simulink model "F250Main"  (R2020b)
settings: Solver=ode8  StartTime=0.0  StopTime=10  FixedStep=0.001  RelTol=1e-3
model workspace: external: MATLAB File C:\Users\zxz\Desktop\matlab\m2020b\F250SimGithub\F250Main_DataFile.m (data not in the file)
values from neighbouring files (symbols this model uses):
  FData = [ 5.1001, ... (first row only)    [F250Main_DataFile.m]
  m = 1.13    [F250Main_DataFile.m]
  PWMData = 0.5:0.05:1    [F250Main_DataFile.m]
undefined symbols (not defined in the file or in its folder): smiData, X, Y, Z
libraries: sm_lib x125, nesl_utility x36, aerolibconvert2 x13, sharedtransform x1
(part 1 of 3)
settings Model: Creator=zxz  LastModifiedBy=zxz

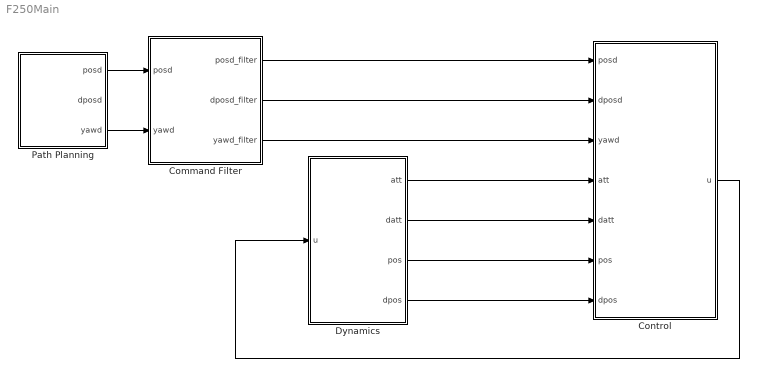
== system F250Main ==
  Command Filter : Subsystem
  Control : Subsystem
  Dynamics : Subsystem
  Path Planning : Subsystem
  wires:
  Path Planning/1(posd) -> Command Filter/1(posd)
  Path Planning/3(yawd) -> Command Filter/2(yawd)
  Control/1(u) -> Dynamics/1(u)
  Command Filter/1(posd_filter) -> Control/1(posd)
  Command Filter/2(dposd_filter) -> Control/2(dposd)
  Command Filter/3(yawd_filter) -> Control/3(yawd)
  Dynamics/1(att) -> Control/4(att)
  Dynamics/2(datt) -> Control/5(datt)
  Dynamics/3(pos) -> Control/6(pos)
  Dynamics/4(dpos) -> Control/7(dpos)

== system F250Main/Command Filter ==
  posd : Inport
  yawd : Inport  Port=2
  Demux11 : Demux  Outputs=3
  Mux1 : Mux  Inputs=3
  Mux8 : Mux  Inputs=3
  X Channel : Subsystem
  Y Channel : Subsystem
  Yaw Channel : Subsystem
  Z Channel : Subsystem
  posd_filter : Outport  VectorParamsAs1DForOutWhenUnconnected=off
  dposd_filter : Outport  Port=2  VectorParamsAs1DForOutWhenUnconnected=off
  yawd_filter : Outport  Port=3  VectorParamsAs1DForOutWhenUnconnected=off
  wires:
  yawd/1 -> Yaw Channel/1(yawd)
  posd/1 -> Demux11/1
  Demux11/1 -> X Channel/1(xd)
  Demux11/2 -> Y Channel/1(yd)
  Demux11/3 -> Z Channel/1(zd)
  Yaw Channel/1(zd_filter) -> yawd_filter/1
  Mux8/1 -> posd_filter/1
  X Channel/1(xd_filter) -> Mux8/1
  Y Channel/1(yd_filter) -> Mux8/2
  Z Channel/1(zd_filter) -> Mux8/3
  X Channel/2(dxd_filter) -> Mux1/1
  Y Channel/2(dyd_filter) -> Mux1/2
  Z Channel/2(dzd_filter) -> Mux1/3
  Mux1/1 -> dposd_filter/1

== system F250Main/Control ==
  posd : Inport
  dposd : Inport  Port=2
  yawd : Inport  Port=3
  att : Inport  Port=4
  datt : Inport  Port=5
  pos : Inport  Port=6
  dpos : Inport  Port=7
  Cascade Attitude Control : Subsystem
  Mux : Mux
  Mux1 : Mux  Inputs=3
  Position Control : Subsystem
  u : Outport  VectorParamsAs1DForOutWhenUnconnected=off
  wires:
  Mux/1 -> u/1
  att/1 -> Position Control/5(att), Cascade Attitude Control/2(att)
  datt/1 -> Cascade Attitude Control/3(datt)
  Mux1/1 -> Cascade Attitude Control/1(attd)
  yawd/1 -> Mux1/3
  Cascade Attitude Control/1(u2) -> Mux/2
  Cascade Attitude Control/2(u3) -> Mux/3
  Cascade Attitude Control/3(u4) -> Mux/4
  posd/1 -> Position Control/1(posd)
  dposd/1 -> Position Control/2(dposd)
  pos/1 -> Position Control/3(pos)
  dpos/1 -> Position Control/4(dpos)
  Position Control/1(u1) -> Mux/1
  Position Control/2(rolld) -> Mux1/1
  Position Control/3(pitchd) -> Mux1/2

== system F250Main/Dynamics ==
  u : Inport
  Infinite Plane : sm_lib/Curves and Surfaces/Infinite Plane  GraphicType=Rectangle  GraphicPlaneWidth=5  GraphicPlaneWidthUnits=m  GraphicPlaneHeight=5  GraphicPlaneHeightUnits=m  GraphicVisPropType=SimpleVisualProperties  GraphicDiffuseColor=[0.5 0.5 0.5]  GraphicOpacity=0.25  GraphicSpecularColor=[0.5 0.5 0.5 1.0]  GraphicAmbientColor=[0.15 0.15 0.15 1.0]  GraphicEmissiveColor=[0.0 0.0 0.0 1.0]  GraphicShininess=75
  MechanismConfiguration : sm_lib/Utilities/Mechanism Configuration  UniformGravity=Constant  GravityVector=[0 0 -9.81]  GravityVectorUnits=m/s^2  GravityUnits=m/s^2  LinearizationDelta=0.001  JointModeTransitionNonlinearIterations=2
  Rigid Transform : sm_lib/Frames and Transforms/Rigid Transform  TranslationMethod=Cartesian  TranslationStandardOffset=0  TranslationLengthUnit=m  TranslationStandardAxis=+Z  TranslationCartesianOffset=[0 0 -0.5]  TranslationROffset=0  TranslationROffsetUnits=m  TranslationZOffset=0  TranslationZOffsetUnits=m  TranslationThetaOffset=0  TranslationThetaOffsetUnits=deg  RotationMethod=None  RotationAngleUnits=deg  RotationStandardAxis=+Z  RotationAngle=0.0  RotationArbitraryAxis=[0 0 1]  FollAlignAxisA=+X  BaseAlignAxisA=+Y  FollAlignAxisB=+Y  BaseAlignAxisB=+Z  RotationSequenceAxes=FollowerAxes  RotationSequence=XYX  RotationSequenceAngles=[0 0 0]  RotationSequenceAnglesUnits=deg  RotationMatrix=[1 0 0; 0 1 0; 0 0 1]
  Solver Configuration : nesl_utility/Solver Configuration  PhysicalDomain=network_engine_domain  SubClassName=solver  LeftPortType=input  RightPortType=generic  Tones=[]  Harmonics=[]  SimulateNoise=off  Profile=off  UseLocalSampling=off  EnableSwitchedLinearOptims=on  FrequencyDomain=off  UseCCode=off  RelTol=0.001  AbsTol=1e-06  MinStep=1e-09  ToWorkspace=off  RevertToSquareIcSolve=off  NumHomotopyIterations=100  PhasorMode=off  PhasorModeNumHarmonics=1  DoDC=off  ResidualTolerance=1e-09  UseLocalSolver=off  LocalSolverChoice=NE_BACKWARD_EULER_ADVANCER  LocalSolverSampleTime=0.001  DoFixedCost=off  MaxNonlinIter=3  MaxModeIter=2  ComputeImpulses=off  ImpulseIterations=2  LinearAlgebra=auto  EquationFormulation=NE_TIME_EF  DelaysMemoryBudget=1024  AutomaticFiltering=on  FilteringTimeConstant=0.001  PartitionStorageMethod=AS_NEEDED  PartitionMemoryBudget=1024  PartitionMethod=ROBUST
  Subsystem : Subsystem
  Transform : sm_lib/Frames and Transforms/Rigid Transform  TranslationMethod=Cartesian  TranslationStandardOffset=0  TranslationLengthUnit=mm  TranslationStandardAxis=+Z  TranslationCartesianOffset=smiData.RigidTransform(4).translation  TranslationROffset=0  TranslationROffsetUnits=m  TranslationZOffset=0  TranslationZOffsetUnits=m  TranslationThetaOffset=0  TranslationThetaOffsetUnits=deg  RotationMethod=ArbitraryAxis  RotationAngleUnits=rad  RotationStandardAxis=+Z  RotationAngle=smiData.RigidTransform(4).angle  RotationArbitraryAxis=smiData.RigidTransform(4).axis  FollAlignAxisA=+X  BaseAlignAxisA=+Y  FollAlignAxisB=+Y  BaseAlignAxisB=+Z  RotationSequenceAxes=FollowerAxes  RotationSequence=XYX  RotationSequenceAngles=[0 0 0]  RotationSequenceAnglesUnits=deg  RotationMatrix=[1 0 0; 0 1 0; 0 0 1]
  World : sm_lib/Frames and Transforms/World Frame
  att : Outport  VectorParamsAs1DForOutWhenUnconnected=off
  datt : Outport  Port=2  VectorParamsAs1DForOutWhenUnconnected=off
  pos : Outport  Port=3  VectorParamsAs1DForOutWhenUnconnected=off
  dpos : Outport  Port=4  VectorParamsAs1DForOutWhenUnconnected=off
  wires:
  Subsystem/4(dpos) -> dpos/1
  Subsystem/3(pos) -> pos/1
  Subsystem/1(att) -> att/1
  Subsystem/2(datt) -> datt/1
  u/1 -> Subsystem/1(u)
  connections:
  Transform/LConn1 -- MechanismConfiguration/RConn1 -- Rigid Transform/LConn1 -- Solver Configuration/RConn1 -- World/RConn1
  Rigid Transform/RConn1 -- Subsystem/LConn2 -- Infinite Plane/LConn1
  Infinite Plane/RConn1 -- Subsystem/LConn3
  Transform/RConn1 -- Subsystem/LConn1

== system F250Main/Path Planning ==
  Constant1 : Constant  Value=0
  Constant10 : Constant  Value=2
  Constant2 : Constant  Value=0
  Constant3 : Constant  Value=0
  Constant7 : Constant  Value=pi/3
  Constant8 : Constant  Value=5
  Constant9 : Constant  Value=2
  Mux3 : Mux  Inputs=3
  Mux4 : Mux  Inputs=3
  posd : Outport
  dposd : Outport  Port=2
  yawd : Outport  Port=3
  wires:
  Constant1/1 -> Mux3/1
  Constant3/1 -> Mux3/3
  Constant2/1 -> Mux3/2
  Constant9/1 -> Mux4/2
  Mux3/1 -> dposd/1
  Constant8/1 -> Mux4/1
  Constant10/1 -> Mux4/3
  Mux4/1 -> posd/1
  Constant7/1 -> yawd/1

== system F250Main/Command Filter/X Channel ==
  xd : Inport
  Derivative : Derivative
  Derivative1 : Derivative
  MATLAB Function : MATLAB Function  TreatAsAtomicUnit=on
  MATLAB Function1 : MATLAB Function  TreatAsAtomicUnit=on
  Memory : Memory
  Memory1 : Memory
  Saturation : Saturate  UpperLimit=2  LowerLimit=-2
  Saturation1 : Saturate  UpperLimit=1  LowerLimit=-1
  Scope1 : Scope  NumInputPorts=2
  Virtual Second Order System : Subsystem
  xd_filter : Outport  VectorParamsAs1DForOutWhenUnconnected=off
  dxd_filter : Outport  Port=2  VectorParamsAs1DForOutWhenUnconnected=off
  wires:
  MATLAB Function/1(vd) -> Saturation/1
  MATLAB Function1/2(e) -> Derivative1/1
  Derivative1/1 -> Memory1/1
  Memory/1 -> MATLAB Function/3(de)
  Virtual Second Order System/1(xd_filter) -> xd_filter/1, MATLAB Function/2(xdnow), Scope1/2  "x"
  xd/1 -> Scope1/1, MATLAB Function/1(xdreal)  "xd"
  MATLAB Function1/1(u) -> Saturation1/1
  Virtual Second Order System/2(dxd_filter) -> dxd_filter/1, MATLAB Function1/2(dxdnow)  "v"
  Saturation1/1 -> Virtual Second Order System/1(xd_u)
  Memory1/1 -> MATLAB Function1/3(de)
  Saturation/1 -> MATLAB Function1/1(dxdreal)  "vd"
  MATLAB Function/2(e) -> Derivative/1
  Derivative/1 -> Memory/1

== system F250Main/Command Filter/Y Channel ==
  yd : Inport
  Derivative : Derivative
  Derivative1 : Derivative
  MATLAB Function : MATLAB Function  TreatAsAtomicUnit=on
  MATLAB Function1 : MATLAB Function  TreatAsAtomicUnit=on
  Memory : Memory
  Memory1 : Memory
  Saturation : Saturate  UpperLimit=2  LowerLimit=-2
  Saturation1 : Saturate  UpperLimit=1  LowerLimit=-1
  Scope1 : Scope  NumInputPorts=2
  Virtual Second Order System : Subsystem
  yd_filter : Outport  VectorParamsAs1DForOutWhenUnconnected=off
  dyd_filter : Outport  Port=2  VectorParamsAs1DForOutWhenUnconnected=off
  wires:
  MATLAB Function/1(vd) -> Saturation/1
  MATLAB Function1/2(e) -> Derivative1/1
  Derivative1/1 -> Memory1/1
  Memory/1 -> MATLAB Function/3(de)
  Virtual Second Order System/1(xd_filter) -> MATLAB Function/2(xdnow), Scope1/2, yd_filter/1  "x"
  yd/1 -> Scope1/1, MATLAB Function/1(xdreal)  "xd"
  MATLAB Function1/1(u) -> Saturation1/1
  Virtual Second Order System/2(dxd_filter) -> dyd_filter/1, MATLAB Function1/2(dxdnow)  "v"
  Saturation1/1 -> Virtual Second Order System/1(xd_u)
  Memory1/1 -> MATLAB Function1/3(de)
  Saturation/1 -> MATLAB Function1/1(dxdreal)  "vd"
  MATLAB Function/2(e) -> Derivative/1
  Derivative/1 -> Memory/1

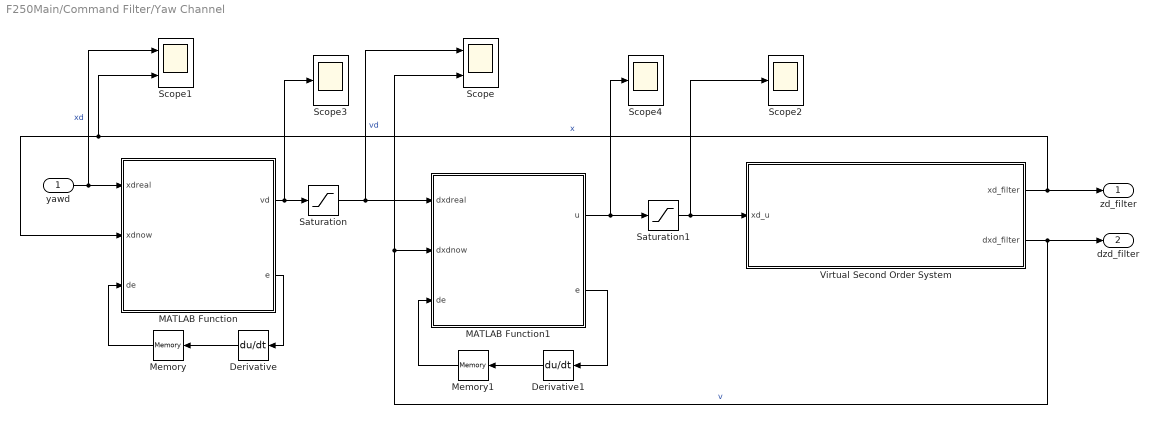
== system F250Main/Command Filter/Yaw Channel ==
  yawd : Inport
  Derivative : Derivative
  Derivative1 : Derivative
  MATLAB Function : MATLAB Function  TreatAsAtomicUnit=on
  MATLAB Function1 : MATLAB Function  TreatAsAtomicUnit=on
  Memory : Memory
  Memory1 : Memory
  Saturation : Saturate  UpperLimit=pi/3  LowerLimit=-pi/3
  Saturation1 : Saturate  UpperLimit=3*pi  LowerLimit=-3*pi
  Scope : Scope  NumInputPorts=2
  Scope1 : Scope  NumInputPorts=2
  Scope2 : Scope
  Scope3 : Scope
  Scope4 : Scope
  Virtual Second Order System : Subsystem
  zd_filter : Outport  VectorParamsAs1DForOutWhenUnconnected=off
  dzd_filter : Outport  Port=2  VectorParamsAs1DForOutWhenUnconnected=off
  wires:
  MATLAB Function/1(vd) -> Scope3/1, Saturation/1
  MATLAB Function1/2(e) -> Derivative1/1
  Derivative1/1 -> Memory1/1
  Memory/1 -> MATLAB Function/3(de)
  Virtual Second Order System/1(xd_filter) -> zd_filter/1, MATLAB Function/2(xdnow), Scope1/2  "x"
  yawd/1 -> Scope1/1, MATLAB Function/1(xdreal)  "xd"
  MATLAB Function1/1(u) -> Scope4/1, Saturation1/1
  Virtual Second Order System/2(dxd_filter) -> dzd_filter/1, Scope/2, MATLAB Function1/2(dxdnow)  "v"
  Saturation1/1 -> Scope2/1, Virtual Second Order System/1(xd_u)
  Memory1/1 -> MATLAB Function1/3(de)
  Saturation/1 -> Scope/1, MATLAB Function1/1(dxdreal)  "vd"
  MATLAB Function/2(e) -> Derivative/1
  Derivative/1 -> Memory/1

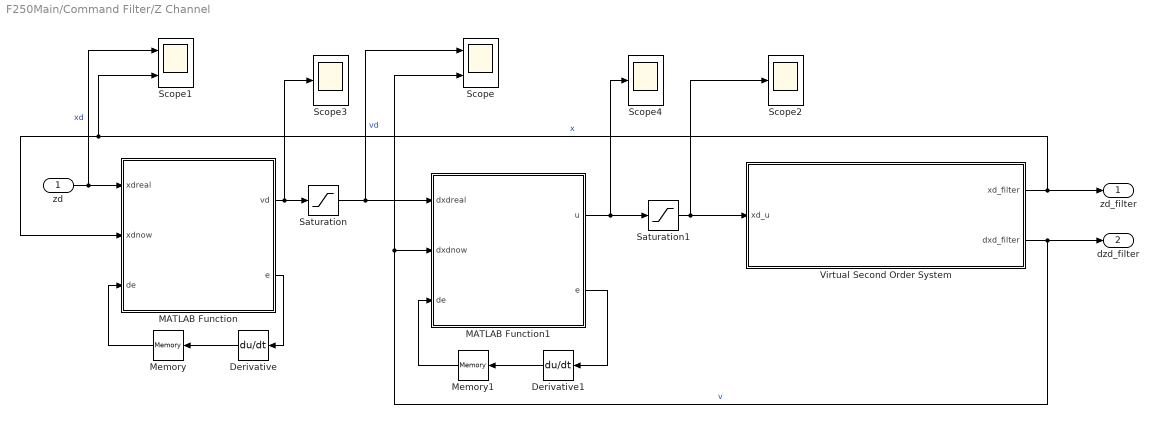
== system F250Main/Command Filter/Z Channel ==
  zd : Inport
  Derivative : Derivative
  Derivative1 : Derivative
  MATLAB Function : MATLAB Function  TreatAsAtomicUnit=on
  MATLAB Function1 : MATLAB Function  TreatAsAtomicUnit=on
  Memory : Memory
  Memory1 : Memory
  Saturation : Saturate  UpperLimit=2  LowerLimit=-2
  Saturation1 : Saturate  UpperLimit=1  LowerLimit=-1
  Scope : Scope  NumInputPorts=2
  Scope1 : Scope  NumInputPorts=2
  Scope2 : Scope
  Scope3 : Scope
  Scope4 : Scope
  Virtual Second Order System : Subsystem
  zd_filter : Outport  VectorParamsAs1DForOutWhenUnconnected=off
  dzd_filter : Outport  Port=2  VectorParamsAs1DForOutWhenUnconnected=off
  wires:
  MATLAB Function/1(vd) -> Scope3/1, Saturation/1
  MATLAB Function1/2(e) -> Derivative1/1
  Derivative1/1 -> Memory1/1
  Memory/1 -> MATLAB Function/3(de)
  Virtual Second Order System/1(xd_filter) -> zd_filter/1, MATLAB Function/2(xdnow), Scope1/2  "x"
  zd/1 -> Scope1/1, MATLAB Function/1(xdreal)  "xd"
  MATLAB Function1/1(u) -> Scope4/1, Saturation1/1
  Virtual Second Order System/2(dxd_filter) -> dzd_filter/1, Scope/2, MATLAB Function1/2(dxdnow)  "v"
  Saturation1/1 -> Scope2/1, Virtual Second Order System/1(xd_u)
  Memory1/1 -> MATLAB Function1/3(de)
  Saturation/1 -> Scope/1, MATLAB Function1/1(dxdreal)  "vd"
  MATLAB Function/2(e) -> Derivative/1
  Derivative/1 -> Memory/1

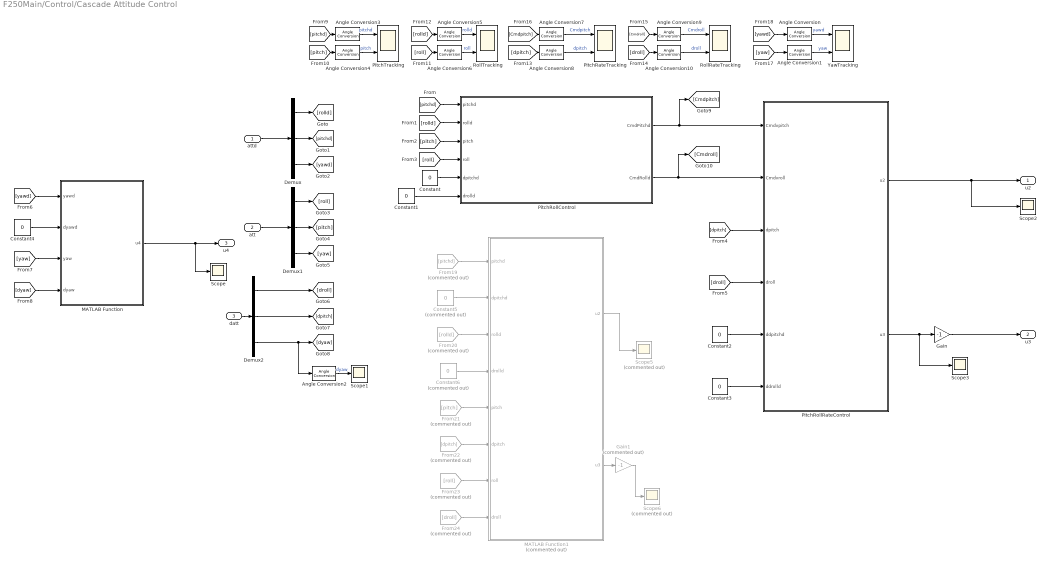
== system F250Main/Control/Cascade Attitude Control ==
  attd : Inport
  att : Inport  Port=2
  datt : Inport  Port=3
  Angle Conversion{,1..10} (11 alike) : aerolibconvert2/Angle Conversion  IU=rad  OU=deg
  Constant{,1..4} (5 alike) : Constant  Value=0
  Constant5 : Constant  Commented=on  Value=0
  Constant6 : Constant  Commented=on  Value=0
  Demux : Demux  Outputs=3
  Demux1 : Demux  Outputs=3
  Demux2 : Demux  Outputs=3
  From19 : From  Commented=on  GotoTag=pitchd
  From20 : From  Commented=on  GotoTag=rolld
  From21 : From  Commented=on  GotoTag=pitch
  From22 : From  Commented=on  GotoTag=dpitch
  From23 : From  Commented=on  GotoTag=roll
  From24 : From  Commented=on  GotoTag=droll
  Gain : Gain  Gain=-1
  Gain1 : Gain  Commented=on  Gain=-1
  MATLAB Function : MATLAB Function  TreatAsAtomicUnit=on
  MATLAB Function1 : MATLAB Function  Commented=on  TreatAsAtomicUnit=on
  PitchRateTracking : Scope  NumInputPorts=2
  PitchRollControl : Subsystem
  PitchRollRateControl : Subsystem
  PitchTracking : Scope  NumInputPorts=2
  RollRateTracking : Scope  NumInputPorts=2
  RollTracking : Scope  NumInputPorts=2
  Scope{,1..3} (4 alike) : Scope
  Scope5 : Scope  Commented=on
  Scope6 : Scope  Commented=on
  YawTracking : Scope  NumInputPorts=2
  u2 : Outport  VectorParamsAs1DForOutWhenUnconnected=off
  u3 : Outport  Port=2  VectorParamsAs1DForOutWhenUnconnected=off
  u4 : Outport  Port=3  VectorParamsAs1DForOutWhenUnconnected=off
  wires:
  attd/1 -> Demux/1
  Demux/1 -> [rolld]
  Demux/2 -> [pitchd]
  Demux/3 -> [yawd]
  Demux1/1 -> [roll]
  Demux1/2 -> [pitch]
  Demux1/3 -> [yaw]
  att/1 -> Demux1/1
  [pitchd] -> PitchRollControl/1(pitchd)
  [rolld] -> PitchRollControl/2(rolld)
  [pitch] -> PitchRollControl/3(pitch)
  [roll] -> PitchRollControl/4(roll)
  Constant1/1 -> PitchRollControl/6(drolld)
  Constant/1 -> PitchRollControl/5(dpitchd)
  [droll] -> PitchRollRateControl/4(droll)
  [dpitch] -> PitchRollRateControl/3(dpitch)
  PitchRollControl/1(CmdPitchd) -> [Cmdpitch], PitchRollRateControl/1(Cmdvpitch)
  PitchRollControl/2(CmdRolld) -> [Cmdroll], PitchRollRateControl/2(Cmdvroll)
  Constant2/1 -> PitchRollRateControl/5(ddpitchd)
  Constant3/1 -> PitchRollRateControl/6(ddrolld)
  [yawd] -> MATLAB Function/1(yawd)
  [yaw] -> MATLAB Function/3(yaw)
  [yawd] -> Angle Conversion/1
  [yaw] -> Angle Conversion1/1
  Angle Conversion/1 -> YawTracking/1  "yawd"
  Angle Conversion1/1 -> YawTracking/2  "yaw"
  Angle Conversion2/1 -> Scope1/1  "dyaw"
  [pitchd] -> Angle Conversion3/1
  Angle Conversion3/1 -> PitchTracking/1  "pitchd"
  [pitch] -> Angle Conversion4/1
  Angle Conversion4/1 -> PitchTracking/2  "pitch"
  [rolld] -> Angle Conversion5/1
  Angle Conversion5/1 -> RollTracking/1  "rolld"
  [roll] -> Angle Conversion6/1
  Angle Conversion6/1 -> RollTracking/2  "roll"
  [Cmdpitch] -> Angle Conversion7/1
  Angle Conversion7/1 -> PitchRateTracking/1  "Cmdpitch"
  Angle Conversion8/1 -> PitchRateTracking/2  "dpitch"
  [dpitch] -> Angle Conversion8/1
  [Cmdroll] -> Angle Conversion9/1
  Angle Conversion9/1 -> RollRateTracking/1  "Cmdroll"
  [droll] -> Angle Conversion10/1
  Angle Conversion10/1 -> RollRateTracking/2  "droll"
  [dyaw] -> MATLAB Function/4(dyaw)
  Constant4/1 -> MATLAB Function/2(dyawd)
  From19/1 -> MATLAB Function1/1(pitchd)
  From20/1 -> MATLAB Function1/3(rolld)
  Constant5/1 -> MATLAB Function1/2(dpitchd)
  Constant6/1 -> MATLAB Function1/4(drolld)
  From21/1 -> MATLAB Function1/5(pitch)
  From22/1 -> MATLAB Function1/6(dpitch)
  From23/1 -> MATLAB Function1/7(roll)
  From24/1 -> MATLAB Function1/8(droll)
  MATLAB Function1/1(u2) -> Scope5/1
  MATLAB Function1/2(u3) -> Gain1/1
  Gain1/1 -> Scope6/1
  MATLAB Function/1(u4) -> Scope/1, u4/1
  PitchRollRateControl/1(u2) -> Scope2/1, u2/1
  Gain/1 -> u3/1
  PitchRollRateControl/2(u3) -> Scope3/1, Gain/1
  datt/1 -> Demux2/1
  Demux2/2 -> [dpitch]
  Demux2/3 -> Angle Conversion2/1, [dyaw]
  Demux2/1 -> [droll]

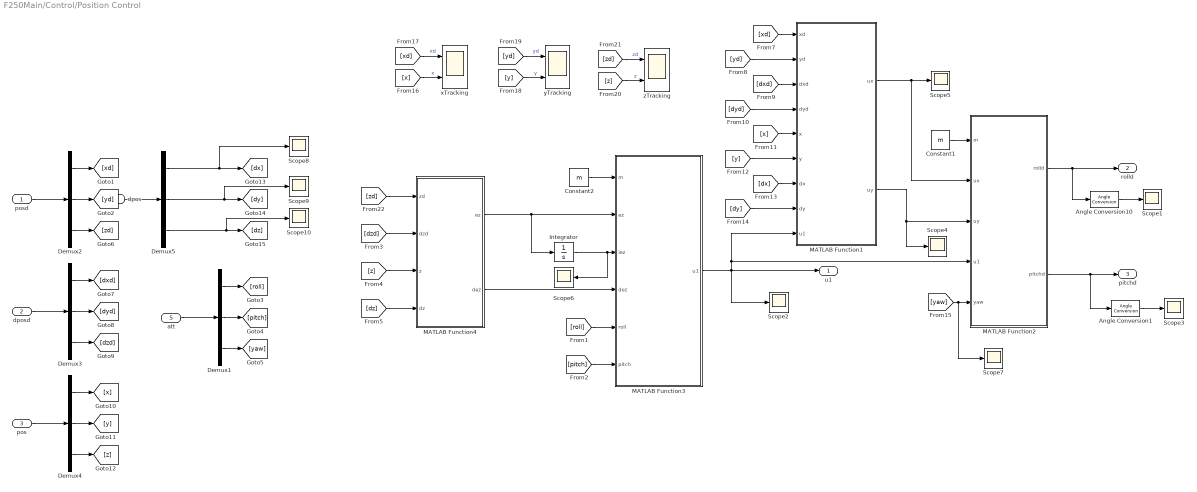
== system F250Main/Control/Position Control ==
  posd : Inport
  dposd : Inport  Port=2
  pos : Inport  Port=3
  dpos : Inport  Port=4
  att : Inport  Port=5
  Angle Conversion1 : aerolibconvert2/Angle Conversion  IU=rad  OU=deg
  Angle Conversion10 : aerolibconvert2/Angle Conversion  IU=rad  OU=deg
  Constant1 : Constant  Value=m
  Constant2 : Constant  Value=m
  Demux{1..5} (5 alike) : Demux  Outputs=3
  Integrator : Integrator
  MATLAB Function1 : MATLAB Function  TreatAsAtomicUnit=on
  MATLAB Function2 : MATLAB Function  TreatAsAtomicUnit=on
  MATLAB Function3 : MATLAB Function  TreatAsAtomicUnit=on
  MATLAB Function4 : MATLAB Function  TreatAsAtomicUnit=on
  Scope{1..10} (10 alike) : Scope
  xTracking : Scope  NumInputPorts=2
  yTracking : Scope  NumInputPorts=2
  zTracking : Scope  NumInputPorts=2
  u1 : Outport  VectorParamsAs1DForOutWhenUnconnected=off
  rolld : Outport  Port=2  VectorParamsAs1DForOutWhenUnconnected=off
  pitchd : Outport  Port=3  VectorParamsAs1DForOutWhenUnconnected=off
  wires:
  att/1 -> Demux1/1
  Demux1/2 -> [pitch]
  Demux1/3 -> [yaw]
  Demux1/1 -> [roll]
  posd/1 -> Demux2/1
  Demux2/1 -> [xd]
  Demux2/3 -> [zd]
  Demux2/2 -> [yd]
  dposd/1 -> Demux3/1
  Demux3/1 -> [dxd]
  Demux3/2 -> [dyd]
  Demux3/3 -> [dzd]
  pos/1 -> Demux4/1
  Demux4/3 -> [z]
  Demux4/2 -> [y]
  Demux4/1 -> [x]
  dpos/1 -> Demux5/1
  MATLAB Function3/1(u1) -> Scope2/1, u1/1, MATLAB Function1/9(u1), MATLAB Function2/4(u1)
  [pitch] -> MATLAB Function3/6(pitch)
  [roll] -> MATLAB Function3/5(roll)
  [xd] -> MATLAB Function1/1(xd)
  [yd] -> MATLAB Function1/2(yd)
  [dxd] -> MATLAB Function1/3(dxd)
  [dyd] -> MATLAB Function1/4(dyd)
  [x] -> MATLAB Function1/5(x)
  [y] -> MATLAB Function1/6(y)
  [dx] -> MATLAB Function1/7(dx)
  [dy] -> MATLAB Function1/8(dy)
  MATLAB Function1/1(ux) -> Scope5/1, MATLAB Function2/2(ux)
  MATLAB Function1/2(uy) -> Scope4/1, MATLAB Function2/3(uy)
  MATLAB Function2/1(rolld) -> Angle Conversion10/1, rolld/1
  [yaw] -> Scope7/1, MATLAB Function2/5(yaw)
  Constant1/1 -> MATLAB Function2/1(m)
  [xd] -> xTracking/1  "xd"
  [x] -> xTracking/2  "x"
  [y] -> yTracking/2  "y"
  [yd] -> yTracking/1  "yd"
  [zd] -> zTracking/1  "zd"
  [z] -> zTracking/2  "z"
  Constant2/1 -> MATLAB Function3/1(m)
  [zd] -> MATLAB Function4/1(zd)
  MATLAB Function4/2(dez) -> MATLAB Function3/4(dez)
  Integrator/1 -> Scope6/1, MATLAB Function3/3(iez)
  MATLAB Function4/1(ez) -> Integrator/1, MATLAB Function3/2(ez)
  [z] -> MATLAB Function4/3(z)
  [dz] -> MATLAB Function4/4(dz)
  [dzd] -> MATLAB Function4/2(dzd)
  Angle Conversion10/1 -> Scope1/1
  Angle Conversion1/1 -> Scope3/1
  MATLAB Function2/2(pitchd) -> Angle Conversion1/1, pitchd/1
  Demux5/1 -> Scope8/1, [dx]
  Demux5/2 -> Scope9/1, [dy]
  Demux5/3 -> Scope10/1, [dz]

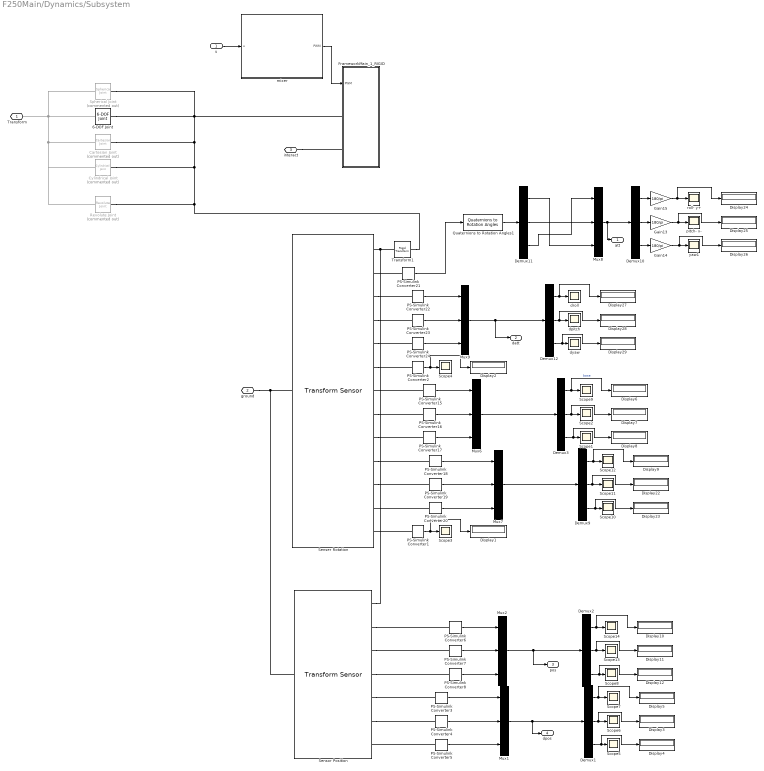
== system F250Main/Dynamics/Subsystem ==
  u : Inport
  6-DOF Joint : sm_lib/Joints/6-DOF Joint  JointMode=Normal  SenseConstraintForce=off  SenseConstraintForceX=off  SenseConstraintForceY=off  SenseConstraintForceZ=off  SenseConstraintTorque=off  SenseConstraintTorqueX=off  SenseConstraintTorqueY=off  SenseConstraintTorqueZ=off  SenseTotalForce=off  SenseTotalForceX=off  SenseTotalForceY=off  SenseTotalForceZ=off  SenseTotalTorque=off  SenseTotalTorqueX=off  SenseTotalTorqueY=off  SenseTotalTorqueZ=off  CompositeWrenchDir=FollowerOnBase  CompositeWrenchFrame=BaseFrame  PxEquilibriumPosition=0  PxEquilibriumPositionUnits=m  PxSpringStiffness=0  PxSpringStiffnessUnits=N/m  PxDampingCoefficient=0  PxDampingCoefficientUnits=N/(m/s)  PxTorqueActuationMode=NoTorque  PxMotionActuationMode=ComputedMotion  PxSensePosition=off  PxSenseVelocity=off  PxSenseAcceleration=off  PxSenseTorqueForce=off  PxSenseLowerLimitTorqueForce=off  PxSenseUpperLimitTorqueForce=off  PxLowerLimitSpecify=off  PxLowerLimitBound=-1  PxLowerLimitBoundUnits=m  PxLowerLimitStiffness=1e6  PxLowerLimitStiffnessUnits=N/m  PxLowerLimitDamping=1e3  PxLowerLimitDampingUnits=N/(m/s)  PxLowerLimitTransitionRegionWidth=1e-4  PxLowerLimitTransitionRegionWidthUnits=m  PxUpperLimitSpecify=off  PxUpperLimitBound=1  PxUpperLimitBoundUnits=m  PxUpperLimitStiffness=1e6  PxUpperLimitStiffnessUnits=N/m  PxUpperLimitDamping=1e3  PxUpperLimitDampingUnits=N/(m/s)  PxUpperLimitTransitionRegionWidth=1e-4  PxUpperLimitTransitionRegionWidthUnits=m  PxPositionTargetSpecify=off  PxPositionTargetPriority=High  PxPositionTargetValue=0  PxPositionTargetValueUnits=m  PxVelocityTargetSpecify=off  PxVelocityTargetPriority=High  PxVelocityTargetValue=0  PxVelocityTargetValueUnits=m/s  PyEquilibriumPosition=0  PyEquilibriumPositionUnits=m  PySpringStiffness=0  PySpringStiffnessUnits=N/m  PyDampingCoefficient=0  PyDampingCoefficientUnits=N/(m/s)  PyTorqueActuationMode=NoTorque  PyMotionActuationMode=ComputedMotion  PySensePosition=off  PySenseVelocity=off  PySenseAcceleration=off  PySenseTorqueForce=off  PySenseLowerLimitTorqueForce=off  PySenseUpperLimitTorqueForce=off  PyLowerLimitSpecify=off  PyLowerLimitBound=-1  PyLowerLimitBoundUnits=m  PyLowerLimitStiffness=1e6  PyLowerLimitStiffnessUnits=N/m  PyLowerLimitDamping=1e3  PyLowerLimitDampingUnits=N/(m/s)  PyLowerLimitTransitionRegionWidth=1e-4  PyLowerLimitTransitionRegionWidthUnits=m  PyUpperLimitSpecify=off  PyUpperLimitBound=1  PyUpperLimitBoundUnits=m  PyUpperLimitStiffness=1e6  PyUpperLimitStiffnessUnits=N/m  PyUpperLimitDamping=1e3  PyUpperLimitDampingUnits=N/(m/s)  PyUpperLimitTransitionRegionWidth=1e-4  PyUpperLimitTransitionRegionWidthUnits=m  PyPositionTargetSpecify=off  PyPositionTargetPriority=High  PyPositionTargetValue=0  PyPositionTargetValueUnits=m  PyVelocityTargetSpecify=off  PyVelocityTargetPriority=High  PyVelocityTargetValue=0  PyVelocityTargetValueUnits=m/s  PzEquilibriumPosition=0  PzEquilibriumPositionUnits=m  PzSpringStiffness=0  PzSpringStiffnessUnits=N/m  PzDampingCoefficient=0  PzDampingCoefficientUnits=N/(m/s)  PzTorqueActuationMode=NoTorque  PzMotionActuationMode=ComputedMotion  PzSensePosition=off  PzSenseVelocity=off  PzSenseAcceleration=off  PzSenseTorqueForce=off  PzSenseLowerLimitTorqueForce=off  PzSenseUpperLimitTorqueForce=off  PzLowerLimitSpecify=off  PzLowerLimitBound=-1  PzLowerLimitBoundUnits=m  PzLowerLimitStiffness=1e6  PzLowerLimitStiffnessUnits=N/m  PzLowerLimitDamping=1e3  PzLowerLimitDampingUnits=N/(m/s)  PzLowerLimitTransitionRegionWidth=1e-4  PzLowerLimitTransitionRegionWidthUnits=m  PzUpperLimitSpecify=off  PzUpperLimitBound=1  PzUpperLimitBoundUnits=m  PzUpperLimitStiffness=1e6  PzUpperLimitStiffnessUnits=N/m  PzUpperLimitDamping=1e3  PzUpperLimitDampingUnits=N/(m/s)  PzUpperLimitTransitionRegionWidth=1e-4  PzUpperLimitTransitionRegionWidthUnits=m  PzPositionTargetSpecify=off  PzPositionTargetPriority=High  PzPositionTargetValue=0  PzPositionTargetValueUnits=m  PzVelocityTargetSpecify=off  PzVelocityTargetPriority=High  PzVelocityTargetValue=0  PzVelocityTargetValueUnits=m/s  SphDefPosRotationMethod=None  SphDefPosRotationAngleUnits=deg  SphDefPosRotationStandardAxis=+Z  SphDefPosRotationAngle=0.0  SphDefPosRotationArbitraryAxis=[0 0 1]  SphDefPosFollAlignAxisA=+X  SphDefPosBaseAlignAxisA=+Y  SphDefPosFollAlignAxisB=+Y  SphDefPosBaseAlignAxisB=+Z  SphDefPosRotationSequenceAxes=FollowerAxes  SphDefPosRotationSequence=XYX  SphDefPosRotationSequenceAngles=[0 0 0]  SphDefPosRotationSequenceAnglesUnits=deg  SphDefPosRotationMatrix=[1 0 0; 0 1 0; 0 0 1]  SphEqPosRotationMethod=None  SphEqPosRotationAngleUnits=deg  SphEqPosRotationStandardAxis=+Z  SphEqPosRotationAngle=0.0  SphEqPosRotationArbitraryAxis=[0 0 1]  SphEqPosFollAlignAxisA=+X  SphEqPosBaseAlignAxisA=+Y  SphEqPosFollAlignAxisB=+Y  SphEqPosBaseAlignAxisB=+Z  SphEqPosRotationSequenceAxes=FollowerAxes  SphEqPosRotationSequence=XYX  SphEqPosRotationSequenceAngles=[0 0 0]  SphEqPosRotationSequenceAnglesUnits=deg  SphEqPosRotationMatrix=[1 0 0; 0 1 0; 0 0 1]  SphSpringStiffness=0  SphSpringStiffnessUnits=N*m/deg  SphDampingCoefficient=0  SphDampingCoefficientUnits=N*m/(deg/s)  SphActuateTorqueX=off  SphActuateTorqueY=off  SphActuateTorqueZ=off  SphActuateTorque=off  SphTorqueActuationMode=NoTorque  SphMotionActuationMode=ComputedMotion  SphActuationFrame=BaseFrame  SphSensePosition=off  SphSenseVelocityX=off  SphSenseVelocityY=off  SphSenseVelocityZ=off  SphSenseVelocity=off  SphSenseAccelerationX=off  SphSenseAccelerationY=off  SphSenseAccelerationZ=off  SphSenseAcceleration=off  SphSenseTorqueX=off  SphSenseTorqueY=off  SphSenseTorqueZ=off  SphSenseTorqueForce=off  SphSenseLowerLimitTorqueMag=off  SphSenseUpperLimitTorqueMag=off  SphSensingFrame=BaseFrame  SphLowerLimitSpecify=off  SphLowerLimitBound=15  SphLowerLimitBoundUnits=deg  SphLowerLimitStiffness=1e4  SphLowerLimitStiffnessUnits=N*m/deg  SphLowerLimitDamping=10  SphLowerLimitDampingUnits=N*m/(deg/s)  SphLowerLimitTransitionRegionWidth=0.1  SphLowerLimitTransitionRegionWidthUnits=deg  SphUpperLimitSpecify=off  SphUpperLimitBound=45  SphUpperLimitBoundUnits=deg  SphUpperLimitStiffness=1e4  SphUpperLimitStiffnessUnits=N*m/deg  SphUpperLimitDamping=10  SphUpperLimitDampingUnits=N*m/(deg/s)  SphUpperLimitTransitionRegionWidth=0.1  SphUpperLimitTransitionRegionWidthUnits=deg  SphPositionTargetRotationMethod=None  SphPositionTargetRotationAngleUnits=deg  SphPositionTargetRotationStandardAxis=+Z  SphPositionTargetRotationAngle=0.0  SphPositionTargetRotationArbitraryAxis=[0 0 1]  SphPositionTargetFollAlignAxisA=+X  SphPositionTargetBaseAlignAxisA=+Y  SphPositionTargetFollAlignAxisB=+Y  SphPositionTargetBaseAlignAxisB=+Z  SphPositionTargetRotationSequenceAxes=FollowerAxes  SphPositionTargetRotationSequence=XYX  SphPositionTargetRotationSequenceAngles=[0 0 0]  SphPositionTargetRotationSequenceAnglesUnits=deg  SphPositionTargetRotationMatrix=[1 0 0; 0 1 0; 0 0 1]  SphPositionTargetSpecify=off  SphPositionTargetPriority=High  SphVelocityTargetValue=[0 0 0]  SphVelocityTargetValueUnits=deg/s  SphVelocityTargetSpecify=off  SphVelocityTargetPriority=High  SphVelocityTargetInFollowerFrame=on
  Cartesian Joint : sm_lib/Joints/Cartesian Joint  Commented=on  JointMode=Normal  SenseConstraintForce=off  SenseConstraintForceX=off  SenseConstraintForceY=off  SenseConstraintForceZ=off  SenseConstraintTorque=off  SenseConstraintTorqueX=off  SenseConstraintTorqueY=off  SenseConstraintTorqueZ=off  SenseTotalForce=off  SenseTotalForceX=off  SenseTotalForceY=off  SenseTotalForceZ=off  SenseTotalTorque=off  SenseTotalTorqueX=off  SenseTotalTorqueY=off  SenseTotalTorqueZ=off  CompositeWrenchDir=FollowerOnBase  CompositeWrenchFrame=BaseFrame  PxEquilibriumPosition=0  PxEquilibriumPositionUnits=m  PxSpringStiffness=0  PxSpringStiffnessUnits=N/m  PxDampingCoefficient=0  PxDampingCoefficientUnits=N/(m/s)  PxTorqueActuationMode=NoTorque  PxMotionActuationMode=ComputedMotion  PxSensePosition=off  PxSenseVelocity=off  PxSenseAcceleration=off  PxSenseTorqueForce=off  PxSenseLowerLimitTorqueForce=off  PxSenseUpperLimitTorqueForce=off  PxLowerLimitSpecify=off  PxLowerLimitBound=-1  PxLowerLimitBoundUnits=m  PxLowerLimitStiffness=1e6  PxLowerLimitStiffnessUnits=N/m  PxLowerLimitDamping=1e3  PxLowerLimitDampingUnits=N/(m/s)  PxLowerLimitTransitionRegionWidth=1e-4  PxLowerLimitTransitionRegionWidthUnits=m  PxUpperLimitSpecify=off  PxUpperLimitBound=1  PxUpperLimitBoundUnits=m  PxUpperLimitStiffness=1e6  PxUpperLimitStiffnessUnits=N/m  PxUpperLimitDamping=1e3  PxUpperLimitDampingUnits=N/(m/s)  PxUpperLimitTransitionRegionWidth=1e-4  PxUpperLimitTransitionRegionWidthUnits=m  PxPositionTargetSpecify=off  PxPositionTargetPriority=High  PxPositionTargetValue=0  PxPositionTargetValueUnits=m  PxVelocityTargetSpecify=off  PxVelocityTargetPriority=High  PxVelocityTargetValue=0  PxVelocityTargetValueUnits=m/s  PyEquilibriumPosition=0  PyEquilibriumPositionUnits=m  PySpringStiffness=0  PySpringStiffnessUnits=N/m  PyDampingCoefficient=0  PyDampingCoefficientUnits=N/(m/s)  PyTorqueActuationMode=NoTorque  PyMotionActuationMode=ComputedMotion  PySensePosition=off  PySenseVelocity=off  PySenseAcceleration=off  PySenseTorqueForce=off  PySenseLowerLimitTorqueForce=off  PySenseUpperLimitTorqueForce=off  PyLowerLimitSpecify=off  PyLowerLimitBound=-1  PyLowerLimitBoundUnits=m  PyLowerLimitStiffness=1e6  PyLowerLimitStiffnessUnits=N/m  PyLowerLimitDamping=1e3  PyLowerLimitDampingUnits=N/(m/s)  PyLowerLimitTransitionRegionWidth=1e-4  PyLowerLimitTransitionRegionWidthUnits=m  PyUpperLimitSpecify=off  PyUpperLimitBound=1  PyUpperLimitBoundUnits=m  PyUpperLimitStiffness=1e6  PyUpperLimitStiffnessUnits=N/m  PyUpperLimitDamping=1e3  PyUpperLimitDampingUnits=N/(m/s)  PyUpperLimitTransitionRegionWidth=1e-4  PyUpperLimitTransitionRegionWidthUnits=m  PyPositionTargetSpecify=off  PyPositionTargetPriority=High  PyPositionTargetValue=0  PyPositionTargetValueUnits=m  PyVelocityTargetSpecify=off  PyVelocityTargetPriority=High  PyVelocityTargetValue=0  PyVelocityTargetValueUnits=m/s  PzEquilibriumPosition=0  PzEquilibriumPositionUnits=m  PzSpringStiffness=0  PzSpringStiffnessUnits=N/m  PzDampingCoefficient=0  PzDampingCoefficientUnits=N/(m/s)  PzTorqueActuationMode=NoTorque  PzMotionActuationMode=ComputedMotion  PzSensePosition=off  PzSenseVelocity=off  PzSenseAcceleration=off  PzSenseTorqueForce=off  PzSenseLowerLimitTorqueForce=off  PzSenseUpperLimitTorqueForce=off  PzLowerLimitSpecify=off  PzLowerLimitBound=-1  PzLowerLimitBoundUnits=m  PzLowerLimitStiffness=1e6  PzLowerLimitStiffnessUnits=N/m  PzLowerLimitDamping=1e3  PzLowerLimitDampingUnits=N/(m/s)  PzLowerLimitTransitionRegionWidth=1e-4  PzLowerLimitTransitionRegionWidthUnits=m  PzUpperLimitSpecify=off  PzUpperLimitBound=1  PzUpperLimitBoundUnits=m  PzUpperLimitStiffness=1e6  PzUpperLimitStiffnessUnits=N/m  PzUpperLimitDamping=1e3  PzUpperLimitDampingUnits=N/(m/s)  PzUpperLimitTransitionRegionWidth=1e-4  PzUpperLimitTransitionRegionWidthUnits=m  PzPositionTargetSpecify=off  PzPositionTargetPriority=High  PzPositionTargetValue=0  PzPositionTargetValueUnits=m  PzVelocityTargetSpecify=off  PzVelocityTargetPriority=High  PzVelocityTargetValue=0  PzVelocityTargetValueUnits=m/s
  Cylindrical Joint : sm_lib/Joints/Cylindrical Joint  Commented=on  JointMode=Normal  SenseConstraintForce=off  SenseConstraintForceX=off  SenseConstraintForceY=off  SenseConstraintForceZ=off  SenseConstraintTorque=off  SenseConstraintTorqueX=off  SenseConstraintTorqueY=off  SenseConstraintTorqueZ=off  SenseTotalForce=off  SenseTotalForceX=off  SenseTotalForceY=off  SenseTotalForceZ=off  SenseTotalTorque=off  SenseTotalTorqueX=off  SenseTotalTorqueY=off  SenseTotalTorqueZ=off  CompositeWrenchDir=FollowerOnBase  CompositeWrenchFrame=BaseFrame  PzEquilibriumPosition=0  PzEquilibriumPositionUnits=m  PzSpringStiffness=0  PzSpringStiffnessUnits=N/m  PzDampingCoefficient=0  PzDampingCoefficientUnits=N/(m/s)  PzTorqueActuationMode=NoTorque  PzMotionActuationMode=ComputedMotion  PzSensePosition=off  PzSenseVelocity=off  PzSenseAcceleration=off  PzSenseTorqueForce=off  PzSenseLowerLimitTorqueForce=off  PzSenseUpperLimitTorqueForce=off  PzLowerLimitSpecify=off  PzLowerLimitBound=-1  PzLowerLimitBoundUnits=m  PzLowerLimitStiffness=1e6  PzLowerLimitStiffnessUnits=N/m  PzLowerLimitDamping=1e3  PzLowerLimitDampingUnits=N/(m/s)  PzLowerLimitTransitionRegionWidth=1e-4  PzLowerLimitTransitionRegionWidthUnits=m  PzUpperLimitSpecify=off  PzUpperLimitBound=1  PzUpperLimitBoundUnits=m  PzUpperLimitStiffness=1e6  PzUpperLimitStiffnessUnits=N/m  PzUpperLimitDamping=1e3  PzUpperLimitDampingUnits=N/(m/s)  PzUpperLimitTransitionRegionWidth=1e-4  PzUpperLimitTransitionRegionWidthUnits=m  PzPositionTargetSpecify=off  PzPositionTargetPriority=High  PzPositionTargetValue=0  PzPositionTargetValueUnits=m  PzVelocityTargetSpecify=off  PzVelocityTargetPriority=High  PzVelocityTargetValue=0  PzVelocityTargetValueUnits=m/s  RzEquilibriumPosition=0  RzEquilibriumPositionUnits=deg  RzSpringStiffness=0  RzSpringStiffnessUnits=N*m/deg  RzDampingCoefficient=0  RzDampingCoefficientUnits=N*m/(deg/s)  RzTorqueActuationMode=NoTorque  RzMotionActuationMode=ComputedMotion  RzSensePosition=off  RzSenseVelocity=off  RzSenseAcceleration=off  RzSenseTorqueForce=off  RzSenseLowerLimitTorqueForce=off  RzSenseUpperLimitTorqueForce=off  RzLowerLimitSpecify=off  RzLowerLimitBound=-90  RzLowerLimitBoundUnits=deg  RzLowerLimitStiffness=1e4  RzLowerLimitStiffnessUnits=N*m/deg  RzLowerLimitDamping=10  RzLowerLimitDampingUnits=N*m/(deg/s)  RzLowerLimitTransitionRegionWidth=0.1  RzLowerLimitTransitionRegionWidthUnits=deg  RzUpperLimitSpecify=off  RzUpperLimitBound=90  RzUpperLimitBoundUnits=deg  RzUpperLimitStiffness=1e4  RzUpperLimitStiffnessUnits=N*m/deg  RzUpperLimitDamping=10  RzUpperLimitDampingUnits=N*m/(deg/s)  RzUpperLimitTransitionRegionWidth=0.1  RzUpperLimitTransitionRegionWidthUnits=deg  RzPositionTargetSpecify=off  RzPositionTargetPriority=High  RzPositionTargetValue=0  RzPositionTargetValueUnits=deg  RzVelocityTargetSpecify=off  RzVelocityTargetPriority=High  RzVelocityTargetValue=0  RzVelocityTargetValueUnits=deg/s
  Demux{1..3,9..12} (7 alike) : Demux  Outputs=3
  Display{1..12,22..29} (20 alike) : Display
  FrameworkMain_1_RIGID : Subsystem
      settings: PortSchema="{\"entries\":[{\"content\":{\"sides\":[{\"content\":{\"connectorIds\":[]},\"type\":\"ConnectorPlacement.EquallySpacedRectSide\",\"uuid\":\"0caf7e8c-9e03-4f5f-a992-e16f2378ddae\"},{\"content\":{\"connectorIds\":[\"In1\",\"RConn1\",\"RConn2\"],\"side\":\"RIGHT\"},\"type\":\"ConnectorPlacement.EquallySpacedRectSide\",\"uuid\":\"c6e5997e-2e06-4849-9791-3be2f1724a0b\"},{\"content\":{\"connectorIds\":[],\"side\":\"TOP\"},\"type\":\"ConnectorPlacement.EquallySpacedRectSide\",\"uuid\":\"d6cd59f4-623c-42f4-a0c8-501115ef4ce2\"},{\"content\":{\"connectorIds\":[],\"side\":\"HIDDEN\"},\"type\":\"ConnectorPlacement.EquallySpacedRectSide\",\"uuid\":\"674c4375-2084-402b-9316-475938a683ce\"}]},\"type\":\"ConnectorPlacement.EquallySpacedConnector\",\"uuid\":\"fbd12e93-a4f1-446f-980d-653a314d83df\"}],\"packageUris\":[\"http://schema.mathworks.com/mf0/Connector/R2020b\"],\"version\":\"1.0\"}"
  Gain13 : Gain  Gain=180/pi
  Gain14 : Gain  Gain=180/pi
  Gain15 : Gain  Gain=180/pi
  Mux{1..2,6..9} (6 alike) : Mux  Inputs=3
  PS-Simulink Converter{1..8,15..24} (18 alike) : nesl_utility/PS-Simulink Converter  PhysicalDomain=network_engine_domain  SubClassName=ps_output  LeftPortType=input  RightPortType=output  PseudoPeriodic=off  Frequencies=[]  Unit=1  AffineConversion=off
  Quaternions to Rotation Angles1 : sharedtransform/Quaternions to Rotation Angles  rotationOrder=ZYX  aMode=aMode
      settings: SourceProductBaseCode=AE
  Revolute Joint : sm_lib/Joints/Revolute Joint  Commented=on  JointMode=Normal  SenseConstraintForce=off  SenseConstraintForceX=off  SenseConstraintForceY=off  SenseConstraintForceZ=off  SenseConstraintTorque=off  SenseConstraintTorqueX=off  SenseConstraintTorqueY=off  SenseConstraintTorqueZ=off  SenseTotalForce=off  SenseTotalForceX=off  SenseTotalForceY=off  SenseTotalForceZ=off  SenseTotalTorque=off  SenseTotalTorqueX=off  SenseTotalTorqueY=off  SenseTotalTorqueZ=off  CompositeWrenchDir=FollowerOnBase  CompositeWrenchFrame=BaseFrame  EquilibriumPosition=0  EquilibriumPositionUnits=deg  SpringStiffness=0  SpringStiffnessUnits=N*m/deg  DampingCoefficient=0  DampingCoefficientUnits=N*m/(deg/s)  TorqueActuationMode=NoTorque  MotionActuationMode=ComputedMotion  SensePosition=off  SenseVelocity=off  SenseAcceleration=off  SenseTorqueForce=off  SenseLowerLimitTorqueForce=off  SenseUpperLimitTorqueForce=off  LowerLimitSpecify=off  LowerLimitBound=-90  LowerLimitBoundUnits=deg  LowerLimitStiffness=1e4  LowerLimitStiffnessUnits=N*m/deg  LowerLimitDamping=10  LowerLimitDampingUnits=N*m/(deg/s)  LowerLimitTransitionRegionWidth=0.1  LowerLimitTransitionRegionWidthUnits=deg  UpperLimitSpecify=off  UpperLimitBound=90  UpperLimitBoundUnits=deg  UpperLimitStiffness=1e4  UpperLimitStiffnessUnits=N*m/deg  UpperLimitDamping=10  UpperLimitDampingUnits=N*m/(deg/s)  UpperLimitTransitionRegionWidth=0.1  UpperLimitTransitionRegionWidthUnits=deg  PositionTargetSpecify=off  PositionTargetPriority=High  PositionTargetValue=0  PositionTargetValueUnits=deg  VelocityTargetSpecify=off  VelocityTargetPriority=High  VelocityTargetValue=0  VelocityTargetValueUnits=deg/s
  Scope{1..14} (14 alike) : Scope
  Senser Rotation : sm_lib/Frames and Transforms/Transform Sensor  MeasurementFrame=Follower  SenseAngle=off  SenseAxis=off  SenseAngle1=off  SenseAngle2=off  SenseAngle3=off  SenseQ=on  SenseR=off  SenseOmegaX=on  SenseOmegaY=on  SenseOmegaZ=on  SenseOmega1=off  SenseOmega2=off  SenseOmega3=off  SenseQDot=off  SenseRDot=off  SenseAlphaX=off  SenseAlphaY=off  SenseAlphaZ=on  SenseAlpha1=off  SenseAlpha2=off  SenseAlpha3=off  SenseQDDot=off  SenseRDDot=off  SenseX=on  SenseY=on  SenseZ=on  SenseRad=off  SenseAzim=off  SenseDist=off  SenseInc=off  SenseXDot=on  SenseYDot=on  SenseZDot=on  SenseRadDot=off  SenseAzimDot=off  SenseDistDot=off  SenseIncDot=off  SenseXDDot=off  SenseYDDot=off  SenseZDDot=on  SenseRadDDot=off  SenseAzimDDot=off  SenseDistDDot=off  SenseIncDDot=off
  Sensor Position : sm_lib/Frames and Transforms/Transform Sensor  MeasurementFrame=World  SenseAngle=off  SenseAxis=off  SenseAngle1=off  SenseAngle2=off  SenseAngle3=off  SenseQ=off  SenseR=off  SenseOmegaX=off  SenseOmegaY=off  SenseOmegaZ=off  SenseOmega1=off  SenseOmega2=off  SenseOmega3=off  SenseQDot=off  SenseRDot=off  SenseAlphaX=off  SenseAlphaY=off  SenseAlphaZ=off  SenseAlpha1=off  SenseAlpha2=off  SenseAlpha3=off  SenseQDDot=off  SenseRDDot=off  SenseX=on  SenseY=on  SenseZ=on  SenseRad=off  SenseAzim=off  SenseDist=off  SenseInc=off  SenseXDot=on  SenseYDot=on  SenseZDot=on  SenseRadDot=off  SenseAzimDot=off  SenseDistDot=off  SenseIncDot=off  SenseXDDot=off  SenseYDDot=off  SenseZDDot=off  SenseRadDDot=off  SenseAzimDDot=off  SenseDistDDot=off  SenseIncDDot=off
  Spherical Joint : sm_lib/Joints/Spherical Joint  Commented=on  JointMode=Normal  SenseConstraintForce=off  SenseConstraintForceX=off  SenseConstraintForceY=off  SenseConstraintForceZ=off  SenseConstraintTorque=off  SenseConstraintTorqueX=off  SenseConstraintTorqueY=off  SenseConstraintTorqueZ=off  SenseTotalForce=off  SenseTotalForceX=off  SenseTotalForceY=off  SenseTotalForceZ=off  SenseTotalTorque=off  SenseTotalTorqueX=off  SenseTotalTorqueY=off  SenseTotalTorqueZ=off  CompositeWrenchDir=FollowerOnBase  CompositeWrenchFrame=BaseFrame  DefPosRotationMethod=None  DefPosRotationAngleUnits=deg  DefPosRotationStandardAxis=+Z  DefPosRotationAngle=0.0  DefPosRotationArbitraryAxis=[0 0 1]  DefPosFollAlignAxisA=+X  DefPosBaseAlignAxisA=+Y  DefPosFollAlignAxisB=+Y  DefPosBaseAlignAxisB=+Z  DefPosRotationSequenceAxes=FollowerAxes  DefPosRotationSequence=XYX  DefPosRotationSequenceAngles=[0 0 0]  DefPosRotationSequenceAnglesUnits=deg  DefPosRotationMatrix=[1 0 0; 0 1 0; 0 0 1]  EqPosRotationMethod=None  EqPosRotationAngleUnits=deg  EqPosRotationStandardAxis=+Z  EqPosRotationAngle=0.0  EqPosRotationArbitraryAxis=[0 0 1]  EqPosFollAlignAxisA=+X  EqPosBaseAlignAxisA=+Y  EqPosFollAlignAxisB=+Y  EqPosBaseAlignAxisB=+Z  EqPosRotationSequenceAxes=FollowerAxes  EqPosRotationSequence=XYX  EqPosRotationSequenceAngles=[0 0 0]  EqPosRotationSequenceAnglesUnits=deg  EqPosRotationMatrix=[1 0 0; 0 1 0; 0 0 1]  SpringStiffness=0  SpringStiffnessUnits=N*m/deg  DampingCoefficient=0  DampingCoefficientUnits=N*m/(deg/s)  ActuateTorqueX=off  ActuateTorqueY=off  ActuateTorqueZ=off  ActuateTorque=off  TorqueActuationMode=NoTorque  MotionActuationMode=ComputedMotion  ActuationFrame=BaseFrame  SensePosition=off  SenseVelocityX=off  SenseVelocityY=off  SenseVelocityZ=off  SenseVelocity=off  SenseAccelerationX=off  SenseAccelerationY=off  SenseAccelerationZ=off  SenseAcceleration=off  SenseTorqueX=off  SenseTorqueY=off  SenseTorqueZ=off  SenseTorqueForce=off  SenseLowerLimitTorqueMag=off  SenseUpperLimitTorqueMag=off  SensingFrame=BaseFrame  LowerLimitSpecify=off  LowerLimitBound=15  LowerLimitBoundUnits=deg  LowerLimitStiffness=1e4  LowerLimitStiffnessUnits=N*m/deg  LowerLimitDamping=10  LowerLimitDampingUnits=N*m/(deg/s)  LowerLimitTransitionRegionWidth=0.1  LowerLimitTransitionRegionWidthUnits=deg  UpperLimitSpecify=off  UpperLimitBound=45  UpperLimitBoundUnits=deg  UpperLimitStiffness=1e4  UpperLimitStiffnessUnits=N*m/deg  UpperLimitDamping=10  UpperLimitDampingUnits=N*m/(deg/s)  UpperLimitTransitionRegionWidth=0.1  UpperLimitTransitionRegionWidthUnits=deg  PositionTargetRotationMethod=None  PositionTargetRotationAngleUnits=deg  PositionTargetRotationStandardAxis=+Z  PositionTargetRotationAngle=0.0  PositionTargetRotationArbitraryAxis=[0 0 1]  PositionTargetFollAlignAxisA=+X  PositionTargetBaseAlignAxisA=+Y  PositionTargetFollAlignAxisB=+Y  PositionTargetBaseAlignAxisB=+Z  PositionTargetRotationSequenceAxes=FollowerAxes  PositionTargetRotationSequence=XYX  PositionTargetRotationSequenceAngles=[0 0 0]  PositionTargetRotationSequenceAnglesUnits=deg  PositionTargetRotationMatrix=[1 0 0; 0 1 0; 0 0 1]  PositionTargetSpecify=off  PositionTargetPriority=High  VelocityTargetValue=[0 0 0]  VelocityTargetValueUnits=deg/s  VelocityTargetSpecify=off  VelocityTargetPriority=High  VelocityTargetInFollowerFrame=on
  Transform1 : sm_lib/Frames and Transforms/Rigid Transform  TranslationMethod=Cartesian  TranslationStandardOffset=0  TranslationLengthUnit=mm  TranslationStandardAxis=+Z  TranslationCartesianOffset=smiData.RigidTransform(4).translation  TranslationROffset=0  TranslationROffsetUnits=m  TranslationZOffset=0  TranslationZOffsetUnits=m  TranslationThetaOffset=0  TranslationThetaOffsetUnits=deg  RotationMethod=ArbitraryAxis  RotationAngleUnits=rad  RotationStandardAxis=+Z  RotationAngle=smiData.RigidTransform(4).angle  RotationArbitraryAxis=smiData.RigidTransform(4).axis  FollAlignAxisA=+X  BaseAlignAxisA=+Y  FollAlignAxisB=+Y  BaseAlignAxisB=+Z  RotationSequenceAxes=FollowerAxes  RotationSequence=XYX  RotationSequenceAngles=[0 0 0]  RotationSequenceAnglesUnits=deg  RotationMatrix=[1 0 0; 0 1 0; 0 0 1]
  dpitch : Scope
  droll : Scope
  dyaw : Scope
  mixer : Subsystem
  pitch- x- : Scope
  roll- y+ : Scope
  yaw1 : Scope
  Transform : PMIOPort  Side=Left
  ground : PMIOPort  Port=2  Side=Left
  interact : PMIOPort  Port=3  Side=Left
  att : Outport  VectorParamsAs1DForOutWhenUnconnected=off
  datt : Outport  Port=2  VectorParamsAs1DForOutWhenUnconnected=off
  pos : Outport  Port=3  VectorParamsAs1DForOutWhenUnconnected=off
  dpos : Outport  Port=4  VectorParamsAs1DForOutWhenUnconnected=off
  wires:
  Demux3/1 -> Display6/1, Scope9/1  "base"
  Mux6/1 -> Demux3/1
  Demux3/3 -> Display8/1, Scope1/1
  Demux3/2 -> Display7/1, Scope2/1
  PS-Simulink Converter16/1 -> Mux6/2
  PS-Simulink Converter15/1 -> Mux6/1
  PS-Simulink Converter19/1 -> Mux7/2
  PS-Simulink Converter18/1 -> Mux7/1
  Demux9/1 -> Display9/1, Scope12/1
  Mux7/1 -> Demux9/1
  Demux9/3 -> Display23/1, Scope10/1
  Demux9/2 -> Display22/1, Scope11/1
  Demux10/1 -> Gain15/1
  Gain14/1 -> Display26/1, yaw1/1
  Demux10/2 -> Gain13/1
  Gain13/1 -> Display25/1, pitch- x-/1
  Quaternions to Rotation Angles1/1 -> Demux11/1
  Demux10/3 -> Gain14/1
  Demux11/1 -> Mux8/3
  Gain15/1 -> Display24/1, roll- y+/1
  Mux8/1 -> att/1, Demux10/1
  PS-Simulink Converter21/1 -> Quaternions to Rotation Angles1/1
  Demux12/3 -> Display29/1, dyaw/1
  Mux9/1 -> datt/1, Demux12/1
  PS-Simulink Converter23/1 -> Mux9/2
  PS-Simulink Converter24/1 -> Mux9/3
  Demux12/1 -> Display27/1, droll/1
  Demux12/2 -> Display28/1, dpitch/1
  PS-Simulink Converter22/1 -> Mux9/1
  u/1 -> mixer/1(u)
  mixer/1(PWM) -> FrameworkMain_1_RIGID/1(PWM)
  PS-Simulink Converter1/1 -> Display1/1, Scope3/1
  PS-Simulink Converter2/1 -> Display2/1, Scope4/1
  PS-Simulink Converter17/1 -> Mux6/3
  PS-Simulink Converter20/1 -> Mux7/3
  Demux11/2 -> Mux8/2
  Demux11/3 -> Mux8/1
  PS-Simulink Converter3/1 -> Mux1/1
  Demux1/3 -> Display4/1, Scope5/1
  Demux1/2 -> Display3/1, Scope6/1
  Mux1/1 -> dpos/1, Demux1/1
  PS-Simulink Converter5/1 -> Mux1/3
  PS-Simulink Converter4/1 -> Mux1/2
  Demux1/1 -> Display5/1, Scope7/1
  Demux2/2 -> Display11/1, Scope13/1
  PS-Simulink Converter6/1 -> Mux2/1
  PS-Simulink Converter8/1 -> Mux2/3
  Demux2/3 -> Display12/1, Scope8/1
  Demux2/1 -> Display10/1, Scope14/1
  Mux2/1 -> pos/1, Demux2/1
  PS-Simulink Converter7/1 -> Mux2/2
  connections:
  Transform1/RConn1 -- Revolute Joint/RConn1 -- Cylindrical Joint/RConn1 -- Cartesian Joint/RConn1 -- Spherical Joint/RConn1 -- FrameworkMain_1_RIGID/RConn1 -- 6-DOF Joint/RConn1
  PS-Simulink Converter21/LConn1 -- Senser Rotation/RConn2
  Senser Rotation/RConn4 -- PS-Simulink Converter23/LConn1
  Senser Rotation/RConn5 -- PS-Simulink Converter24/LConn1
  Senser Rotation/RConn3 -- PS-Simulink Converter22/LConn1
  Cartesian Joint/LConn1 -- Revolute Joint/LConn1 -- Cylindrical Joint/LConn1 -- Spherical Joint/LConn1 -- 6-DOF Joint/LConn1 -- Transform/RConn1
  PS-Simulink Converter1/LConn1 -- Senser Rotation/RConn13
  PS-Simulink Converter20/LConn1 -- Senser Rotation/RConn12
  Senser Rotation/RConn11 -- PS-Simulink Converter19/LConn1
  Senser Rotation/RConn10 -- PS-Simulink Converter18/LConn1
  PS-Simulink Converter15/LConn1 -- Senser Rotation/RConn7
  Senser Rotation/RConn8 -- PS-Simulink Converter16/LConn1
  Senser Rotation/RConn9 -- PS-Simulink Converter17/LConn1
  Senser Rotation/RConn6 -- PS-Simulink Converter2/LConn1
  interact/RConn1 -- FrameworkMain_1_RIGID/RConn2
  ground/RConn1 -- Sensor Position/LConn1 -- Senser Rotation/LConn1
  Transform1/LConn1 -- Sensor Position/RConn1 -- Senser Rotation/RConn1
  PS-Simulink Converter5/LConn1 -- Sensor Position/RConn7
  Sensor Position/RConn6 -- PS-Simulink Converter4/LConn1
  Sensor Position/RConn5 -- PS-Simulink Converter3/LConn1
  Sensor Position/RConn4 -- PS-Simulink Converter8/LConn1
  Sensor Position/RConn3 -- PS-Simulink Converter7/LConn1
  Sensor Position/RConn2 -- PS-Simulink Converter6/LConn1

== system F250Main/Command Filter/X Channel/Virtual Second Order System ==
  xd_u : Inport
  Constant1 : Constant  Value=0
  Constant2 : Constant  Value=0
  Integrator : Integrator  InitialConditionSource=external
  Integrator1 : Integrator  InitialConditionSource=external
  xd_filter : Outport
  dxd_filter : Outport  Port=2
  wires:
  Constant1/1 -> Integrator1/2
  Integrator/1 -> dxd_filter/1, Integrator1/1
  Constant2/1 -> Integrator/2
  xd_u/1 -> Integrator/1
  Integrator1/1 -> xd_filter/1

== system F250Main/Command Filter/Y Channel/Virtual Second Order System ==
  xd_u : Inport
  Constant1 : Constant  Value=0
  Constant2 : Constant  Value=0
  Integrator : Integrator  InitialConditionSource=external
  Integrator1 : Integrator  InitialConditionSource=external
  xd_filter : Outport
  dxd_filter : Outport  Port=2
  wires:
  Constant1/1 -> Integrator1/2
  Integrator/1 -> dxd_filter/1, Integrator1/1
  Constant2/1 -> Integrator/2
  xd_u/1 -> Integrator/1
  Integrator1/1 -> xd_filter/1

== system F250Main/Command Filter/Yaw Channel/Virtual Second Order System ==
  xd_u : Inport
  Constant1 : Constant  Value=0
  Constant2 : Constant  Value=0
  Integrator : Integrator  InitialConditionSource=external
  Integrator1 : Integrator  InitialConditionSource=external
  xd_filter : Outport
  dxd_filter : Outport  Port=2
  wires:
  Constant1/1 -> Integrator1/2
  Integrator/1 -> dxd_filter/1, Integrator1/1
  Constant2/1 -> Integrator/2
  xd_u/1 -> Integrator/1
  Integrator1/1 -> xd_filter/1

== system F250Main/Command Filter/Z Channel/Virtual Second Order System ==
  xd_u : Inport
  Constant1 : Constant  Value=0.5
  Constant2 : Constant  Value=0
  Integrator : Integrator  InitialConditionSource=external
  Integrator1 : Integrator  InitialConditionSource=external
  xd_filter : Outport
  dxd_filter : Outport  Port=2
  wires:
  Constant1/1 -> Integrator1/2
  Integrator/1 -> dxd_filter/1, Integrator1/1
  Constant2/1 -> Integrator/2
  xd_u/1 -> Integrator/1
  Integrator1/1 -> xd_filter/1

== system F250Main/Control/Cascade Attitude Control/PitchRollControl ==
  pitchd : Inport
  rolld : Inport  Port=2
  pitch : Inport  Port=3
  roll : Inport  Port=4
  dpitchd : Inport  Port=5
  drolld : Inport  Port=6
  Integrator : Integrator
  Integrator1 : Integrator
  MATLAB Function1 : MATLAB Function  TreatAsAtomicUnit=on
  MATLAB Function3 : MATLAB Function  TreatAsAtomicUnit=on
  Scope4 : Scope
  CmdPitchd : Outport
  CmdRolld : Outport  Port=2
  wires:
  MATLAB Function3/1(epitch) -> Integrator/1, MATLAB Function1/3(epitch)
  pitch/1 -> MATLAB Function3/3(pitch)
  MATLAB Function1/1(CmdPitchd) -> CmdPitchd/1
  roll/1 -> MATLAB Function3/4(roll)
  MATLAB Function1/2(CmdRolld) -> CmdRolld/1
  MATLAB Function3/2(eroll) -> Integrator1/1, MATLAB Function1/4(eroll)
  pitchd/1 -> MATLAB Function3/1(pitchd)
  rolld/1 -> MATLAB Function3/2(rolld)
  Integrator/1 -> Scope4/1, MATLAB Function1/5(eipitch)
  Integrator1/1 -> MATLAB Function1/6(eiroll)
  drolld/1 -> MATLAB Function1/2(drolld)
  dpitchd/1 -> MATLAB Function1/1(dpitchd)
